simulink model "MC_INIT"  (R2023b)
settings: Solver=VariableStepAuto  StartTime=0.0  StopTime=10.0  RelTol=1e-3
settings Model: Creator=rebek  LastModifiedBy=rebek

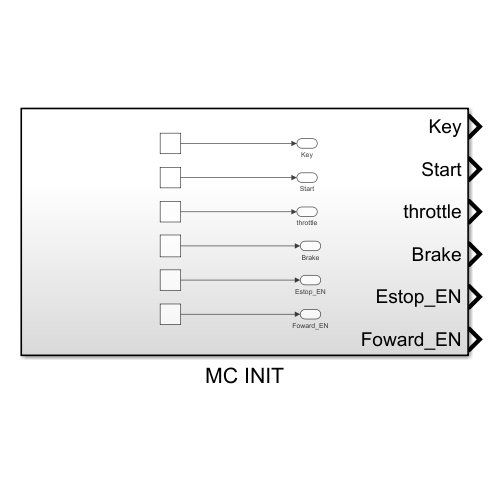
[thumbnail: Simulink's stored preview of the top-level diagram]
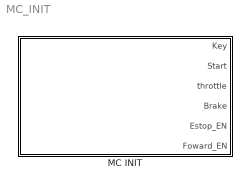
== system MC_INIT ==
  MC INIT : Subsystem

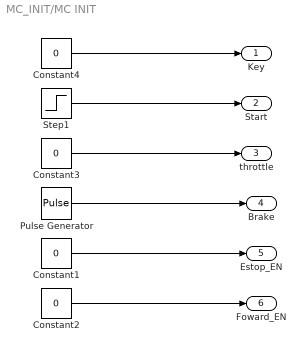
== system MC_INIT/MC INIT ==
  Constant{1..4} (4 alike) : Constant  Value=0
  Pulse Generator : DiscretePulseGenerator  PulseType=Time based  Period=100  PulseWidth=50
  Step1 : Step  Time=200  SampleTime=0
  Key : Outport
  Start : Outport  Port=2
  throttle : Outport  Port=3
  Brake : Outport  Port=4
  Estop_EN : Outport  Port=5
  Foward_EN : Outport  Port=6
  wires:
  Constant4/1 -> Key/1
  Step1/1 -> Start/1
  Constant3/1 -> throttle/1
  Pulse Generator/1 -> Brake/1
  Constant1/1 -> Estop_EN/1
  Constant2/1 -> Foward_EN/1
